simulink model "q1"  (R2020b)
settings: Solver=VariableStepAuto  StartTime=0.0  StopTime=100.0  MaxStep=0.001  RelTol=1e-3
settings Model: Creator=Ravi  LastModifiedBy=Ravi

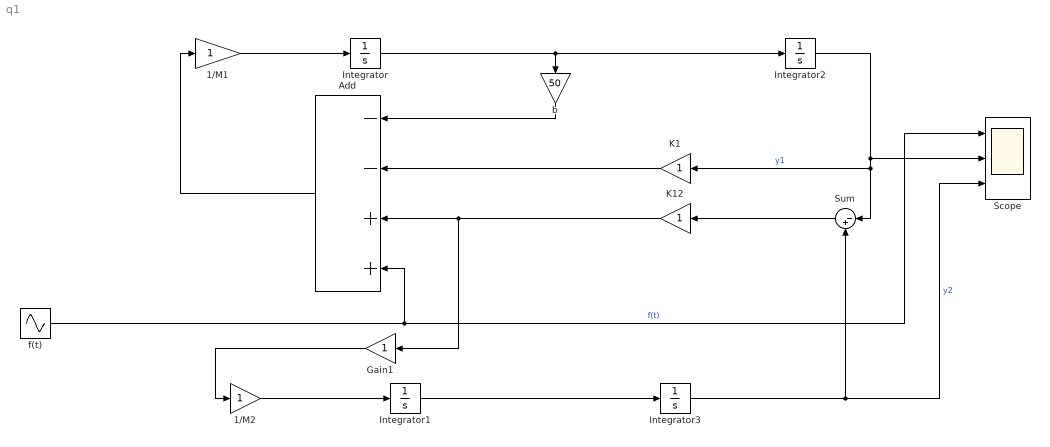
== system q1 ==
  1/M1 : Gain
  1/M2 : Gain
  Add : Sum  Inputs=--++
  Gain1 : Gain
  Integrator{,1..3} (4 alike) : Integrator
  K1 : Gain
  K12 : Gain
  Scope : Scope  NumInputPorts=3
  Sum : Sum  Inputs=|-+
  b : Gain  Gain=50
  f(t) : Sin  Amplitude=2  Frequency=10  SampleTime=0
  wires:
  Add/1 -> 1/M1/1
  1/M1/1 -> Integrator/1
  Integrator/1 -> b/1, Integrator2/1
  b/1 -> Add/1
  K1/1 -> Add/2
  K12/1 -> Gain1/1, Add/3
  Gain1/1 -> 1/M2/1
  f(t)/1 -> Add/4, Scope/1  "f(t)"
  Integrator2/1 -> K1/1, Sum/1, Scope/2  "y1"
  Sum/1 -> K12/1
  Integrator3/1 -> Scope/3, Sum/2  "y2"
  Integrator1/1 -> Integrator3/1
  1/M2/1 -> Integrator1/1
